simulink model "robot2"  (Simulink 7.1)
settings: Solver=ode45  StartTime=0.0  StopTime=10.0  RelTol=1e-3
undefined symbols (not defined in the file): Ts
libraries: mwblocks x37
settings Model: Creator=Bob  LastModifiedBy=Bob
settings OptimizationCC: BooleanDataType=off
settings DebuggingCC: SaveWithParameterizedLinksMsg=none  SignalResolutionControl=TryResolveAllWithWarning  SolverPrmCheckMsg=none  MultiTaskDSMMsg=warning  MultiTaskCondExecSysMsg=none  StrictBusMsg=None
settings HardwareCC: TargetUnknown=on
settings RTWCC: IncludeERTFirstTime=on
settings GRTTargetCC: TargetFcnLib=ansi_tfl_tmw.mat  ModelReferenceCompliant=off  MatFileLogging=off

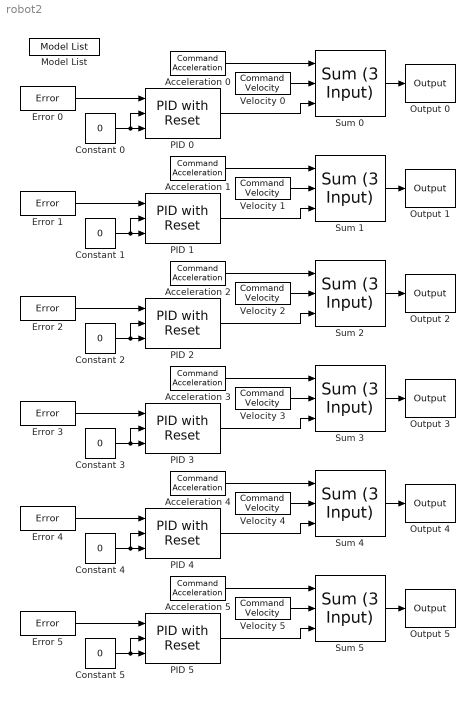
== system robot2 ==
  Acceleration 0 : mwblocks/Command Acceleration  Tag=TCACCEL  SystemSampleTime=-1  meiAxis=6  SubSample=0  User0=0  User1=0
  Acceleration 1 : mwblocks/Command Acceleration  Tag=TCACCEL  SystemSampleTime=-1  meiAxis=7  SubSample=0  User0=0  User1=0
  Acceleration 2 : mwblocks/Command Acceleration  Tag=TCACCEL  SystemSampleTime=-1  meiAxis=8  SubSample=0  User0=0  User1=0
  Acceleration 3 : mwblocks/Command Acceleration  Tag=TCACCEL  SystemSampleTime=-1  meiAxis=9  SubSample=0  User0=0  User1=0
  Acceleration 4 : mwblocks/Command Acceleration  Tag=TCACCEL  SystemSampleTime=-1  meiAxis=10  SubSample=0  User0=0  User1=0
  Acceleration 5 : mwblocks/Command Acceleration  Tag=TCACCEL  SystemSampleTime=-1  meiAxis=11  SubSample=0  User0=0  User1=0
  Constant {0..5} (6 alike) : Constant  Tag=CONSTANT  Value=0  OutDataType=sfix(16)  OutScaling=2^0
  Error 0 : mwblocks/Error  Tag=ERROR  SystemSampleTime=-1  meiAxis=6  SubSample=0  User0=0  User1=0
  Error 1 : mwblocks/Error  Tag=ERROR  SystemSampleTime=-1  meiAxis=7  SubSample=0  User0=0  User1=0
  Error 2 : mwblocks/Error  Tag=ERROR  SystemSampleTime=-1  meiAxis=8  SubSample=0  User0=0  User1=0
  Error 3 : mwblocks/Error  Tag=ERROR  SystemSampleTime=-1  meiAxis=9  SubSample=0  User0=0  User1=0
  Error 4 : mwblocks/Error  Tag=ERROR  SystemSampleTime=-1  meiAxis=10  SubSample=0  User0=0  User1=0
  Error 5 : mwblocks/Error  Tag=ERROR  SystemSampleTime=-1  meiAxis=11  SubSample=0  User0=0  User1=0
  Model List : mwblocks/Model List  Tag=MODEL_LIST  Description=List of model numbers to load this model  SystemSampleTime=-1  meiModelList=1
  Output 0 : mwblocks/Output   Tag=OUTPUT  SystemSampleTime=-1  meiMotor=6  SubSample=0  User0=0  User1=0
  Output 1 : mwblocks/Output   Tag=OUTPUT  SystemSampleTime=-1  meiMotor=7  SubSample=0  User0=0  User1=0
  Output 2 : mwblocks/Output   Tag=OUTPUT  SystemSampleTime=-1  meiMotor=8  SubSample=0  User0=0  User1=0
  Output 3 : mwblocks/Output   Tag=OUTPUT  SystemSampleTime=-1  meiMotor=9  SubSample=0  User0=0  User1=0
  Output 4 : mwblocks/Output   Tag=OUTPUT  SystemSampleTime=-1  meiMotor=10  SubSample=0  User0=0  User1=0
  Output 5 : mwblocks/Output   Tag=OUTPUT  SystemSampleTime=-1  meiMotor=11  SubSample=0  User0=0  User1=0
  PID {0..5} (6 alike) : mwblocks/PID with Reset  Tag=PID_R  Description=PID with integration limit and derivative smoothing.  SystemSampleTime=-1  Kp=0.1  Ki=0  Kd=1.0  Ksm=0  Imax=0  Ts=Ts  SubSample=0  User0=0  User1=0
  Sum 0 : mwblocks/Sum (3 Input)  Tag=SUM  Description=3 Input sum with gains on each input  SystemSampleTime=-1  K1=125  K2=.15  K3=1  SubSample=0  User0=0  User1=0
  Sum 1 : mwblocks/Sum (3 Input)  Tag=SUM  Description=3 Input sum with gains on each input  SystemSampleTime=-1  K1=125  K2=.15  K3=1  SubSample=0  User0=0  User1=0
  Sum 2 : mwblocks/Sum (3 Input)  Tag=SUM  Description=3 Input sum with gains on each input  SystemSampleTime=-1  K1=50  K2=.05  K3=1  SubSample=0  User0=0  User1=0
  Sum 3 : mwblocks/Sum (3 Input)  Tag=SUM  Description=3 Input sum with gains on each input  SystemSampleTime=-1  K1=0  K2=.05  K3=1  SubSample=0  User0=0  User1=0
  Sum 4 : mwblocks/Sum (3 Input)  Tag=SUM  Description=3 Input sum with gains on each input  SystemSampleTime=-1  K1=30  K2=0.4  K3=1  SubSample=0  User0=0  User1=0
  Sum 5 : mwblocks/Sum (3 Input)  Tag=SUM  Description=3 Input sum with gains on each input  SystemSampleTime=-1  K1=0  K2=.05  K3=1  SubSample=0  User0=0  User1=0
  Velocity 0 : mwblocks/Command Velocity  Tag=TCVEL  SystemSampleTime=-1  meiAxis=6  SubSample=0  User0=0  User1=0
  Velocity 1 : mwblocks/Command Velocity  Tag=TCVEL  SystemSampleTime=-1  meiAxis=7  SubSample=0  User0=0  User1=0
  Velocity 2 : mwblocks/Command Velocity  Tag=TCVEL  SystemSampleTime=-1  meiAxis=8  SubSample=0  User0=0  User1=0
  Velocity 3 : mwblocks/Command Velocity  Tag=TCVEL  SystemSampleTime=-1  meiAxis=9  SubSample=0  User0=0  User1=0
  Velocity 4 : mwblocks/Command Velocity  Tag=TCVEL  SystemSampleTime=-1  meiAxis=10  SubSample=0  User0=0  User1=0
  Velocity 5 : mwblocks/Command Velocity  Tag=TCVEL  SystemSampleTime=-1  meiAxis=11  SubSample=0  User0=0  User1=0
  wires:
  Error 0/1 -> PID 0/1
  Sum 0/1 -> Output 0/1
  PID 0/1 -> Sum 0/3
  Acceleration 0/1 -> Sum 0/1
  Velocity 0/1 -> Sum 0/2
  Constant 0/1 -> PID 0/3, PID 0/2
  Error 1/1 -> PID 1/1
  Sum 1/1 -> Output 1/1
  PID 1/1 -> Sum 1/3
  Acceleration 1/1 -> Sum 1/1
  Velocity 1/1 -> Sum 1/2
  Constant 1/1 -> PID 1/3, PID 1/2
  Error 2/1 -> PID 2/1
  Sum 2/1 -> Output 2/1
  PID 2/1 -> Sum 2/3
  Acceleration 2/1 -> Sum 2/1
  Velocity 2/1 -> Sum 2/2
  Constant 2/1 -> PID 2/3, PID 2/2
  Error 3/1 -> PID 3/1
  Sum 3/1 -> Output 3/1
  PID 3/1 -> Sum 3/3
  Acceleration 3/1 -> Sum 3/1
  Velocity 3/1 -> Sum 3/2
  Constant 3/1 -> PID 3/3, PID 3/2
  Error 4/1 -> PID 4/1
  Sum 4/1 -> Output 4/1
  PID 4/1 -> Sum 4/3
  Acceleration 4/1 -> Sum 4/1
  Velocity 4/1 -> Sum 4/2
  Constant 4/1 -> PID 4/3, PID 4/2
  Error 5/1 -> PID 5/1
  Sum 5/1 -> Output 5/1
  PID 5/1 -> Sum 5/3
  Acceleration 5/1 -> Sum 5/1
  Velocity 5/1 -> Sum 5/2
  Constant 5/1 -> PID 5/3, PID 5/2
